simulink model "bignonlinearmodel"  (R2015a)
settings: Solver=ode3  StartTime=0.0  StopTime=10.0  RelTol=1e-3
values from neighbouring files (symbols this model uses):
  g = 9.81    [controlmodeltestspoleplacment.m]    (also in controlwithintegratorsLQR.m; controlwithoutencoderonlyMPUgains.m)
  L = 0.080    (= 0.08)    [controlmodeltestspoleplacment.m]    (also in controlwithintegratorsLQR.m = 0.11; controlwithoutencoderonlyMPUgains.m = 0.068)
  m = (y(:,2)./r)-y(:,4)    [controlwithintegratorsLQR.m]
  R = 5.6/48    (= 0.116666666667)    [controlmodeltestspoleplacment.m]    (also in controlwithintegratorsLQR.m; controlwithoutencoderonlyMPUgains.m)
undefined symbols (not defined in the file or in its folder): fm_l, fm_r, J_eps, J_phi, Jw_l, Jw_r, Kb_l, Kb_r, Kt_l, Kt_r, M, n, R_a, W
settings Model: Creator=omaRhagrass  LastModifiedBy=omaRhagrass
settings SolverCC: PositivePriorityOrder=on  AutoInsertRateTranBlk=on
settings OptimizationCC: InlineParams=on  BufferReuse=off
settings DebuggingCC: InitInArrayFormatMsg=none

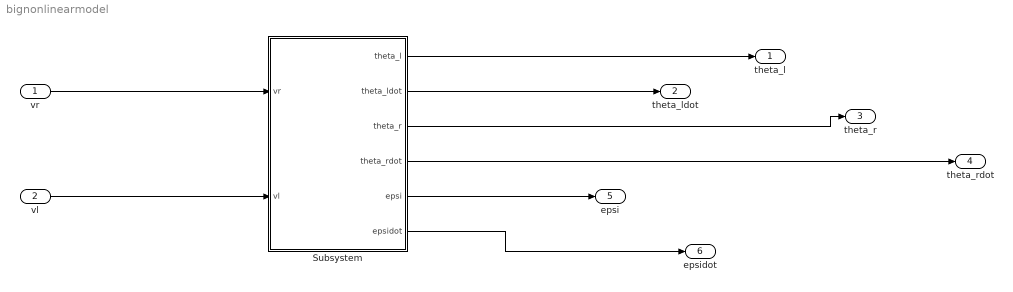
== system bignonlinearmodel ==
  vr : Inport
  "vl " : Inport  Port=2
  Subsystem : Subsystem
  "theta_l " : Outport
  "theta_ldot " : Outport  Port=2
  "theta_r " : Outport  Port=3
  "theta_rdot " : Outport  Port=4
  "epsi " : Outport  Port=5
  "epsidot " : Outport  Port=6
  wires:
  vr/1 -> Subsystem/1(vr)
  "vl "/1 -> Subsystem/2("vl ")
  Subsystem/1("theta_l ") -> "theta_l "/1
  Subsystem/2("theta_ldot ") -> "theta_ldot "/1
  Subsystem/3("theta_r ") -> "theta_r "/1
  Subsystem/4("theta_rdot ") -> "theta_rdot "/1
  Subsystem/5("epsi ") -> "epsi "/1
  Subsystem/6("epsidot ") -> "epsidot "/1

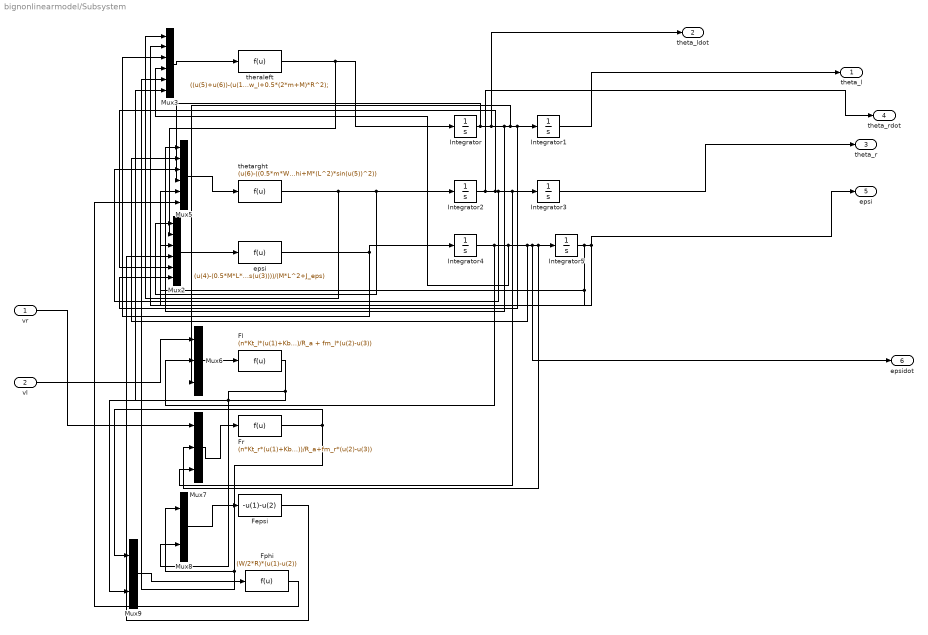
== system bignonlinearmodel/Subsystem ==
  vr : Inport
  "vl " : Inport  Port=2
  Fepsi : Fcn  Expr=-u(1)-u(2)
  Fl : Fcn  Expr=(n*Kt_l*(u(1)+Kb_l*(u(2)-u(3))*n))/R_a + fm_l*(u(2)-u(3))
  "Fphi " : Fcn  Expr=(W/2*R)*(u(1)-u(2))
  "Fr " : Fcn  Expr=(n*Kt_r*(u(1)+Kb_r*(u(2)-u(3))*n))/R_a+fm_r*(u(2)-u(3))
  Integrator{,1..5} (6 alike) : Integrator
  Mux2 : Mux  Inputs=6
  Mux3 : Mux  Inputs=6
  Mux5 : Mux  Inputs=6
  Mux6 : Mux  Inputs=3
  Mux7 : Mux  Inputs=3
  Mux8 : Mux  Inputs=2
  Mux9 : Mux  Inputs=2
  epsi : Fcn  Expr=(u(4)-(0.5*M*L*R*cos(u(3))*(u(1)+u(2))-M*g*L*sin(u(3))-M*(L^2)*((R/W)*(u(5)-u(6)))^2*sin(u(3))*cos(u(3))))/(M*L^2+J_eps)
  "theraleft " : Fcn  Expr=((u(5)+u(6))-(u(1)*0.5*(2*m+M)*(R^2)+Jw_r*u(1)+(M*L*R*cos(u(2)))*u(3)-M*L*R*u(4)^2*sin(u(2))))/(Jw_l+0.5*(2*m+M)*R^2);
  thetarght : Fcn  Expr=(u(6)-((0.5*m*W^2+J_phi+M*(L^2)*sin(u(5))^2)*(R/W)*-u(1)-(W/2*R)*Jw_l*u(1)+2*M*L^2*u(2)*(R/W)*(u(3)-u(4))*sin(u(5))*cos(u(5))))/((W/(2*R))*Jw_r+(R/W)*(0.5*m*W^2+J_phi+M*(L^2)*sin(u(5))^2))
  "theta_l " : Outport
  "theta_ldot " : Outport  Port=2
  "theta_r " : Outport  Port=3
  "theta_rdot " : Outport  Port=4
  "epsi " : Outport  Port=5
  "epsidot " : Outport  Port=6
  wires:
  Integrator1/1 -> "theta_l "/1
  "Fphi "/1 -> Mux5/6
  "theraleft "/1 -> Mux2/2, Integrator/1
  Integrator4/1 -> Mux6/2, Mux5/2, "epsidot "/1, Mux7/2, Integrator5/1, Mux3/4
  "vl "/1 -> Mux6/1
  Integrator5/1 -> Mux5/5, Mux2/3, "epsi "/1, Mux3/2
  Integrator/1 -> Mux5/4, "theta_ldot "/1, Mux5/1, Mux2/6, Integrator1/1, Mux6/3
  Integrator2/1 -> "theta_rdot "/1, Mux2/5, Mux5/3, Integrator3/1, Mux7/3
  Mux7/1 -> "Fr "/1
  Mux9/1 -> "Fphi "/1
  Integrator3/1 -> "theta_r "/1
  Mux8/1 -> Fepsi/1
  Mux3/1 -> "theraleft "/1
  epsi/1 -> Mux3/3, Integrator4/1
  Mux6/1 -> Fl/1
  Mux2/1 -> epsi/1
  thetarght/1 -> Mux3/1, Mux2/1, Integrator2/1
  Fl/1 -> Mux9/2, Mux3/6, Mux8/2
  "Fr "/1 -> Mux3/5, Mux8/1, Mux9/1
  Fepsi/1 -> Mux2/4
  vr/1 -> Mux7/1
  Mux5/1 -> thetarght/1
